simulink model "DCMotor"  (R2024a)
settings: Solver=VariableStepAuto  StartTime=0.0  StopTime=10.0  RelTol=1e-3
values from neighbouring files (symbols this model uses):
  A = zeros(n, n)    [Model1numericalPSA.m]    (also in MotorSens2.m = A_func(x0s,u0,p_sym,z0); Parameter.m = A_func(x0s,u0,z0); Sensitivitaetsanalyse.m = A_func(x0s,u0,z0))
  b = b_func(x0s,u0,p_sym,z0)    [MotorSens2.m]    (also in Parameter.m = b_func(x0s,u0,z0); Sensitivitaetsanalyse.m = b_func(x0s,u0,z0))
  c = c_func(x0s,u0,p_sym,z0)    [MotorSens2.m]    (also in Parameter.m = c_func(x0s,u0,z0); Sensitivitaetsanalyse.m = c_func(x0s,u0,z0))
settings Model: Creator=jakob  LastModifiedBy=jakob

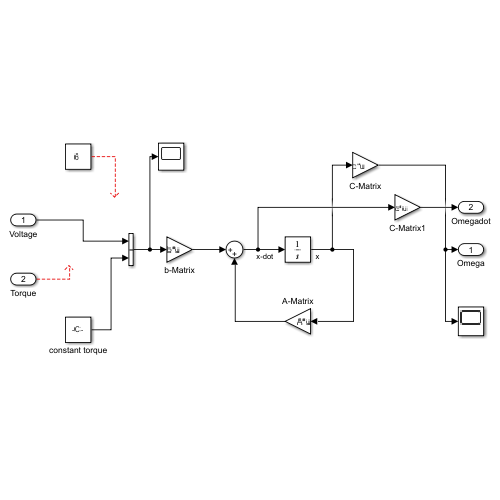
[thumbnail: Simulink's stored preview of the top-level diagram]
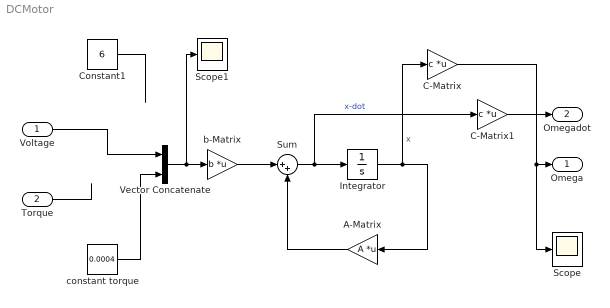
== system DCMotor ==
  Voltage : Inport
  Torque : Inport  Port=2
  A-Matrix : Gain  Gain=A  Multiplication=Matrix(K*u)
  C-Matrix : Gain  Gain=c  Multiplication=Matrix(K*u)
  C-Matrix1 : Gain  Gain=c  Multiplication=Matrix(K*u)
  Constant1 : Constant  Value=6
  Integrator : Integrator
  Scope : Scope
  Scope1 : Scope
  Sum : Sum  Inputs=|++
  Vector Concatenate : Concatenate
  b-Matrix : Gain  Gain=b  Multiplication=Matrix(K*u)
  constant torque : Constant  Value=0.0004
  Omega : Outport
  Omegadot : Outport  Port=2
  wires:
  Voltage/1 -> Vector Concatenate/1
  Torque/1 -> ?
  Vector Concatenate/1 -> Scope1/1, b-Matrix/1
  b-Matrix/1 -> Sum/1
  Sum/1 -> C-Matrix1/1, Integrator/1  "x-dot"
  A-Matrix/1 -> Sum/2
  Integrator/1 -> A-Matrix/1, C-Matrix/1  "x"
  C-Matrix/1 -> Scope/1, Omega/1
  C-Matrix1/1 -> Omegadot/1
  constant torque/1 -> Vector Concatenate/2
  Constant1/1 -> ?
